simulink model "gm_sampleModel66206_pp_7_1_sub"  (R2023b)
settings: Solver=VariableStepAuto  StartTime=0.0  StopTime=10.0  RelTol=1e-3
libraries: simulink x38, hdlsllib x2, hdlmdlgenlib x2
(part 1 of 2)
settings Model: Creator=CW  LastModifiedBy=CW
settings OptimizationCC: BlockReduction=off  ConditionallyExecuteInputs=off
settings DebuggingCC: ArtificialAlgebraicLoopMsg=none  InheritedTsInSrcMsg=none

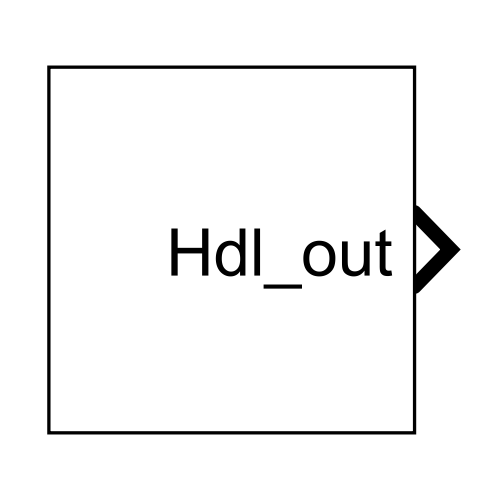
[thumbnail: Simulink's stored preview of the top-level diagram]
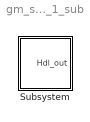
== system gm_sampleModel66206_pp_7_1_sub ==
  Subsystem : Subsystem

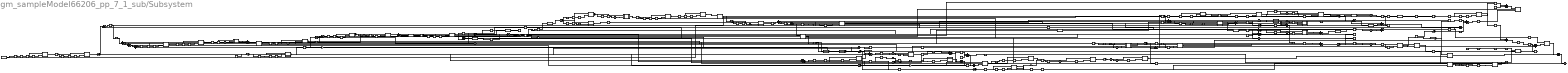
== system gm_sampleModel66206_pp_7_1_sub/Subsystem ==
  Reshape{,1..5} (6 alike) : Reshape
  cfblk1 : Subsystem  mask(Detect Fall Nonpositive){vinit=double(0), InputProcessing=Elements as channels (sample based), OutDataTypeStr=uint8}
      mask prompts: vinit "Simulink:masks:InitialCondition_MP"; InputProcessing "Simulink:masks:InputProcessing_MP"; OutDataTypeStr "Simulink:masks:OutputDataType_MP"
      mask help: Simulink:masks:DetectFallNonpositive_MD
      mask init:
      | InputProcessing = 'Elements as channels (sample based)';
      | OutDataTypeStr = 'uint8';
      | vinit = double(0);
      mask TypeOptions InputProcessing: Simulink:masks:ColumnsAsChannelsFrameBased | Simulink:masks:ElementsAsChannelsSampleBased
      mask TypeOptions OutDataTypeStr: Simulink:masks:uint8 | Simulink:masks:boolean
      mask Display: fprintf('U <= 0\n&  NOT\nU/z <= 0')
  cfblk10 : Subsystem  mask(Detect Rise Positive){vinit=double(0), InputProcessing=Elements as channels (sample based), OutDataTypeStr=uint8}
      mask prompts: vinit "Simulink:masks:InitialCondition_MP"; InputProcessing "Simulink:masks:InputProcessing_MP"; OutDataTypeStr "Simulink:masks:OutputDataType_MP"
      mask help: Simulink:masks:DetectRisePositive_MD
      mask init:
      | InputProcessing = 'Elements as channels (sample based)';
      | OutDataTypeStr = 'uint8';
      | vinit = double(0);
      mask TypeOptions InputProcessing: Simulink:masks:ColumnsAsChannelsFrameBased | Simulink:masks:ElementsAsChannelsSampleBased
      mask TypeOptions OutDataTypeStr: Simulink:masks:uint8 | Simulink:masks:boolean
      mask Display: fprintf('U > 0\n&  NOT\nU/z > 0')
  cfblk{15,22,25,48,52,58,61,63,68,71,90,98..100,106,113,115,118,129,134} (20 alike) : Sum  OutDataTypeStr=uint8  AccumDataTypeStr=uint8  SampleTime=1
  cfblk101 : Subsystem
  cfblk102_inst : Subsystem
  cfblk{29,37,41,46,67,76,93,103,116} (9 alike) : Sum  Inputs=+-  OutDataTypeStr=uint8  AccumDataTypeStr=uint8  SampleTime=1
  cfblk{16,33..34,73,82,91,97,105,121} (9 alike) : Gain  Gain="fi(0,0,8,7,\"hex\",\"80\")"  ParamDataTypeStr=fixdt(0, 8, 7)  OutDataTypeStr=uint8  SampleTime=1
  cfblk{18,79,107,109,125,140..141} (7 alike) : Product  Inputs=*/  OutDataTypeStr=uint8  RndMeth=Zero  SaturateOnIntegerOverflow=on  SampleTime=1
  cfblk108 : Subsystem
  cfblk11 : Subsystem  mask(Detect Fall Nonpositive){vinit=double(0), InputProcessing=Elements as channels (sample based), OutDataTypeStr=uint8}
      mask prompts: vinit "Simulink:masks:InitialCondition_MP"; InputProcessing "Simulink:masks:InputProcessing_MP"; OutDataTypeStr "Simulink:masks:OutputDataType_MP"
      mask help: Simulink:masks:DetectFallNonpositive_MD
      mask init:
      | InputProcessing = 'Elements as channels (sample based)';
      | OutDataTypeStr = 'uint8';
      | vinit = double(0);
      mask TypeOptions InputProcessing: Simulink:masks:ColumnsAsChannelsFrameBased | Simulink:masks:ElementsAsChannelsSampleBased
      mask TypeOptions OutDataTypeStr: Simulink:masks:uint8 | Simulink:masks:boolean
      mask Display: fprintf('U <= 0\n&  NOT\nU/z <= 0')
  cfblk{17,23,38..39,81,83,110,119,132} (9 alike) : ComplexToRealImag  SampleTime=1
  cfblk111 : Subsystem  mask(Real World Value Increment){}
      mask help: Simulink:masks:RealWorldValueIncrement_MD
      mask Display: disp('V++')
  cfblk{49,53,75,89,112,120,133} (7 alike) : Signum  SampleTime=1
  cfblk{60,69,85,114} (4 alike) : Sum  OutDataTypeStr=uint8  AccumDataTypeStr=uint8  RndMeth=Nearest  SampleTime=1
  cfblk114_const_val : Constant  Value=0  VectorParams1D=off  OutDataTypeStr=uint8  SampleTime=1
  cfblk117 : Subsystem
  cfblk12 : RelationalOperator  Operator=<=  OutDataTypeStr=fixdt(0,8,0)  SampleTime=1  InputSameDT=off
  cfblk122 : MinMax  OutDataTypeStr=uint8
  cfblk123 : Subsystem
  cfblk{56,65,124,139} (4 alike) : Abs  SampleTime=1  OutDataTypeStr=uint8  SaturateOnIntegerOverflow=off
  cfblk126 : MinMax  OutDataTypeStr=uint8
  cfblk{64,88,95,127,137} (5 alike) : Sum  Inputs=+  OutDataTypeStr=uint8
  cfblk128_inst : Subsystem
  cfblk13 : Subsystem
  cfblk130 : Subsystem
  cfblk131_inst : Subsystem
  cfblk135_inst : Subsystem
  cfblk136 : Subsystem
  cfblk138 : Subsystem
  cfblk14 : Subsystem
  cfblk143 : Constant  Value=0  VectorParams1D=off  OutDataTypeStr=uint8  SampleTime=1
  cfblk144 : Constant  Value=0  VectorParams1D=off  OutDataTypeStr=uint8  SampleTime=1
  cfblk145 : hdlsllib/Sources/HDL Counter  CountType=Count limited  CountInit=0  CountStep=1  CountMax=25  CountFromType=Initial value  CountFrom=0  CountResetPort=off  CountLoadPort=off  CountEnbPort=off  CountDirPort=off  CountHitOutputPort=off  CountDataType=Unsigned  CountWordLen=8  CountFracLen=0  CountSampTime=1
  cfblk146 : Subsystem
  cfblk147 : Subsystem
  cfblk148 : Subsystem
  cfblk149 : Subsystem
  cfblk150 : Subsystem
  cfblk151 : Subsystem
  cfblk{152..155} (4 alike) : Switch  Threshold=double(0)  OutDataTypeStr=uint8  SampleTime=1  SaturateOnIntegerOverflow=off  InputSameDT=off
  cfblk{156..167,169..174} (18 alike) : Delay  DelayLength=double(2)  InitialCondition=0  SampleTime=1
  cfblk168 : Subsystem
  cfblk{175..179,182..189,191,194..198} (19 alike) : DataTypeConversion  OutDataTypeStr=fixdt(0,8,0)
  cfblk180 : Subsystem
  cfblk181 : Subsystem
  cfblk19 : Subsystem  mask(Real World Value Increment){}
      mask help: Simulink:masks:RealWorldValueIncrement_MD
      mask Display: disp('V++')
  cfblk190 : Subsystem
  cfblk192 : Subsystem
  cfblk193 : Subsystem
  cfblk2 : Subsystem
  cfblk20_inst : Subsystem
  cfblk21 : Subsystem
  cfblk24 : Subsystem
  cfblk26 : Subsystem
  cfblk27 : Subsystem
  cfblk28 : Subsystem
  cfblk3 : RelationalOperator  Operator=<=  OutDataTypeStr=fixdt(0,8,0)  SampleTime=1  InputSameDT=off
  cfblk30_inst : Subsystem
  cfblk32 : Subsystem
  cfblk35 : Subsystem
  cfblk36_inst : Subsystem
  cfblk4 : hdlmdlgenlib/Buffer
  cfblk40 : Subsystem  mask(Real World Value Increment){}
      mask help: Simulink:masks:RealWorldValueIncrement_MD
      mask Display: disp('V++')
  cfblk42_inst : Subsystem
  cfblk44_inst : Subsystem
  cfblk47 : Subsystem
  cfblk5 : Subsystem
  cfblk50 : Subsystem
  cfblk51 : Subsystem
  cfblk54 : Subsystem
  cfblk55 : Subsystem
  cfblk59 : Subsystem  mask(Real World Value Increment){}
      mask help: Simulink:masks:RealWorldValueIncrement_MD
      mask Display: disp('V++')
  cfblk6 : hdlsllib/Logic and Bit Operations/Bit Reduce  mode=AND
  cfblk60_const_val : Constant  Value=0  VectorParams1D=off  OutDataTypeStr=uint8  SampleTime=1
  cfblk66 : Sum  Inputs=+-  OutDataTypeStr=uint8  AccumDataTypeStr=int32  SampleTime=1
  cfblk69_const_val : Constant  Value=0  VectorParams1D=off  OutDataTypeStr=uint8  SampleTime=1
  cfblk7 : hdlmdlgenlib/Buffer
  cfblk70 : Subsystem
  cfblk72 : Subsystem
  cfblk74 : Subsystem
  cfblk77 : Sum  OutDataTypeStr=uint8  AccumDataTypeStr=fixdt(0, 32, 7)  SampleTime=1
  cfblk8 : simulink/Logic and Bit Operations/Bit Set  iBit=double(0)
  cfblk80 : Subsystem  mask(Real World Value Increment){}
      mask help: Simulink:masks:RealWorldValueIncrement_MD
      mask Display: disp('V++')
  cfblk84 : Subsystem
  cfblk85_const_val : Constant  Value=0  VectorParams1D=off  OutDataTypeStr=uint8  SampleTime=1
  cfblk87 : MinMax  OutDataTypeStr=uint8
  cfblk9 : simulink/Logic and Bit Operations/Detect Decrease  vinit=0.0  OutDataTypeStr=uint8
      settings: LibrarySourceBlock=|
      | hdlsllib/Logic and Bit
      | Operations/Detect
      | Decrease
  cfblk92 : Subsystem
  cfblk94_inst : Subsystem
  cfblk96 : Subsystem
  compare{,4,6..7,10..12,15..16,18,20,24..34} (22 alike) : simulink/Logic and Bit Operations/Compare To Constant  relop=>=  const=0  OutDataTypeStr=boolean
  compare{1,5,8,13..14,19,22} (7 alike) : simulink/Logic and Bit Operations/Compare To Constant  relop=>=  const=255  OutDataTypeStr=boolean
  compare{2..3,9,17,21,23} (6 alike) : simulink/Logic and Bit Operations/Compare To Constant  relop=>=  const=1  OutDataTypeStr=boolean
  emi_{7,15,23,31,39,47,55,63,71,79,87,95,103,111,119,127,135,143,151,159,175,183,191,199,215,223,232,240,249,257,265,273,281,289} (34 alike) : DataTypeConversion  OutDataTypeStr=fixdt(0,8,0)
  emi_{8,24,32,40,48,56,64,72,80,88,96,104,136,144,152,184,192,200,224,241,258,290} (22 alike) : Delay  DelayLength=double(2)  InitialCondition=0  SampleTime=1
  emi_{16,112,160,208,216,250,274} (7 alike) : Delay  DelayLength=double(2)  InitialCondition=255  SampleTime=1
  emi_{120,128,176,233,266,282} (6 alike) : Delay  DelayLength=double(2)  InitialCondition=1  SampleTime=1
  emi_207 : DataTypeConversion  OutDataTypeStr=uint8  SampleTime=1  SaturateOnIntegerOverflow=off  RndMeth=Floor
  Hdl_out : Outport  OutDataTypeStr=uint8  SampleTime=1
  wires:
  cfblk1/1(Y) -> cfblk198/1
  cfblk10/1(Y) -> cfblk83/1
  cfblk100/1 -> emi_16/1, cfblk117/1(emi_10)
  cfblk101/1(emi_67) -> emi_88/1, cfblk84/1(emi_82)
  cfblk102_inst/1(out1) -> cfblk66/1, cfblk134/2
  cfblk103/1 -> emi_290/1, cfblk96/1(emi_284)
  Reshape/1 -> cfblk155/3, emi_192/1, cfblk47/1(emi_186)
  cfblk105/1 -> cfblk155/1
  cfblk106/1 -> cfblk76/1
  cfblk107/1 -> emi_64/1, cfblk14/1(emi_58)
  cfblk108/1(emi_2) -> cfblk49/1
  cfblk108/2(emi_3) -> cfblk97/1
  cfblk109/1 -> cfblk166/1
  cfblk11/1(Y) -> cfblk157/1
  cfblk110/1 -> cfblk56/1
  cfblk110/2 -> cfblk48/1
  cfblk111/1(y) -> cfblk89/1
  cfblk112/1 -> emi_48/1, cfblk136/1(emi_42)
  cfblk113/1 -> cfblk153/3, cfblk135_inst/1(in1)
  cfblk114/1 -> emi_250/1, cfblk70/1(emi_243)
  cfblk115/1 -> cfblk134/1
  cfblk116/1 -> cfblk19/1(u)
  cfblk117/1(emi_11) -> cfblk37/1
  cfblk118/1 -> cfblk184/1
  cfblk119/1 -> cfblk73/1
  cfblk119/2 -> cfblk132/1
  cfblk12/1 -> cfblk179/1
  cfblk120/1 -> cfblk63/1, cfblk161/1
  cfblk121/1 -> cfblk186/1, cfblk141/2
  cfblk122/1 -> cfblk11/1(U)
  cfblk123/1(emi_19) -> cfblk77/1
  cfblk124/1 -> cfblk60/1, cfblk100/2, cfblk165/1
  cfblk125/1 -> cfblk116/1, cfblk10/1(U)
  cfblk126/1 -> cfblk195/1
  cfblk127/1 -> cfblk90/1
  cfblk128_inst/1(out1) -> cfblk81/1
  cfblk129/1 -> cfblk163/1
  cfblk13/1(emi_27) -> cfblk113/1
  cfblk130/1(emi_35) -> cfblk53/1
  cfblk131_inst/1(out1) -> cfblk22/2
  cfblk132/1 -> cfblk80/1(u)
  cfblk132/2 -> cfblk167/1
  cfblk133/1 -> cfblk188/1, cfblk174/1
  cfblk134/1 -> emi_72/1, cfblk101/1(emi_66)
  cfblk135_inst/1(out1) -> emi_136/1, cfblk24/1(emi_130)
  cfblk136/1(emi_43) -> Reshape2/1, cfblk41/2
  cfblk137/1 -> cfblk93/2, emi_56/1, cfblk138/1(emi_50)
  cfblk138/1(emi_51) -> cfblk61/2
  cfblk139/1 -> Reshape4/1, cfblk105/1
  cfblk14/1(emi_59) -> cfblk15/2
  cfblk140/1 -> emi_112/1, cfblk192/1(emi_106)
  cfblk141/1 -> cfblk185/1
  cfblk143/1 -> cfblk196/1, cfblk34/1
  cfblk144/1 -> cfblk182/1
  cfblk145/1 -> Reshape/1
  cfblk146/1(Out1) -> cfblk112/1
  cfblk147/1(Out1) -> cfblk175/1
  cfblk148/1(Out1) -> cfblk40/1(u), cfblk64/1
  cfblk149/1(Out1) -> cfblk124/1
  cfblk15/1 -> cfblk158/1
  cfblk150/1(Out1) -> cfblk58/1
  cfblk151/1(Out1) -> cfblk110/1
  cfblk152/1 -> cfblk102_inst/2(in2)
  cfblk153/1 -> cfblk68/2, cfblk122/1
  cfblk154/1 -> cfblk103/2
  cfblk155/1 -> cfblk12/2
  cfblk156/1 -> cfblk116/2
  cfblk157/1 -> cfblk153/2
  cfblk158/1 -> cfblk115/2
  cfblk159/1 -> cfblk152/2
  cfblk16/1 -> cfblk68/1, cfblk67/1
  cfblk160/1 -> cfblk113/2
  cfblk161/1 -> cfblk135_inst/2(in2)
  cfblk162/1 -> cfblk41/1
  cfblk163/1 -> cfblk76/2
  cfblk164/1 -> cfblk141/1
  cfblk165/1 -> cfblk67/2
  cfblk166/1 -> cfblk61/1
  cfblk167/1 -> cfblk71/1
  cfblk168/1(emi_91) -> cfblk125/1
  cfblk169/1 -> cfblk152/3
  cfblk17/1 -> cfblk121/1
  cfblk17/2 -> cfblk9/1
  cfblk170/1 -> cfblk154/2
  cfblk171/1 -> cfblk106/2
  cfblk172/1 -> cfblk20_inst/1(in1)
  cfblk173/1 -> cfblk128_inst/2(in2)
  cfblk174/1 -> cfblk1/1(U)
  cfblk175/1 -> emi_282/1, emi_176/1, cfblk92/1(emi_276), cfblk32/1(emi_170)
  cfblk176/1 -> cfblk147/1(In1)
  cfblk177/1 -> cfblk120/1
  cfblk178/1 -> cfblk99/1
  cfblk179/1 -> cfblk99/2
  cfblk18/1 -> emi_274/1, cfblk181/1(emi_268)
  cfblk180/1(emi_75) -> cfblk93/1, cfblk131_inst/2(in2), cfblk160/1
  cfblk181/1(emi_269) -> cfblk91/1
  cfblk182/1 -> cfblk8/1
  cfblk183/1 -> cfblk102_inst/1(in1)
  cfblk184/1 -> cfblk30_inst/2(in2)
  cfblk185/1 -> cfblk118/1
  cfblk186/1 -> cfblk118/2
  cfblk187/1 -> cfblk75/1
  cfblk188/1 -> cfblk59/1(u)
  cfblk189/1 -> cfblk44_inst/1(in1)
  cfblk19/1(y) -> cfblk71/2
  cfblk190/1(emi_99) -> cfblk25/1
  cfblk191/1 -> cfblk25/2
  cfblk192/1(emi_107) -> emi_160/1, cfblk28/1(emi_154)
  cfblk193/1(emi_115) -> cfblk140/1
  cfblk194/1 -> cfblk140/2
  cfblk195/1 -> cfblk107/1
  cfblk196/1 -> cfblk126/1
  cfblk197/1 -> emi_266/1, cfblk74/1(emi_260)
  cfblk198/1 -> emi_224/1, cfblk51/1(emi_218)
  cfblk2/1(emi_195) -> cfblk18/1
  cfblk20_inst/1(out1) -> emi_184/1, cfblk35/1(emi_178)
  cfblk21/1(emi_123) -> Reshape5/1
  cfblk22/1 -> cfblk162/1
  cfblk23/1 -> cfblk29/2
  cfblk23/2 -> cfblk69/1
  cfblk24/1(emi_131) -> cfblk154/3, cfblk95/1
  cfblk25/1 -> cfblk189/1
  cfblk26/1(emi_139) -> cfblk137/1
  cfblk27/1(emi_147) -> cfblk129/1
  cfblk28/1(emi_155) -> cfblk36_inst/1(in1)
  cfblk29/1 -> cfblk146/1(In1)
  cfblk3/1 -> cfblk176/1
  cfblk30_inst/1(out1) -> cfblk154/1
  cfblk32/1(emi_171) -> cfblk164/1
  cfblk33/1 -> cfblk12/1
  cfblk34/1 -> cfblk94_inst/1(in1)
  cfblk35/1(emi_179) -> cfblk152/1
  cfblk36_inst/1(out1) -> Reshape1/1
  cfblk37/1 -> cfblk111/1(u)
  cfblk38/1 -> cfblk88/1
  cfblk38/2 -> cfblk194/1, cfblk173/1
  cfblk39/1 -> cfblk33/1
  cfblk39/2 -> cfblk3/1
  cfblk4/1 -> cfblk6/1, cfblk125/2
  cfblk40/1(y) -> cfblk65/1, cfblk155/2
  cfblk41/1 -> cfblk153/1, cfblk170/1, cfblk151/1(In1)
  cfblk42_inst/1(out1) -> cfblk172/1
  cfblk44_inst/1(out1) -> cfblk22/1
  Reshape1/1 -> emi_40/1, cfblk130/1(emi_34)
  cfblk46/1 -> cfblk39/1
  cfblk47/1(emi_187) -> cfblk98/2, cfblk63/2, cfblk139/1
  cfblk48/1 -> cfblk46/1
  cfblk49/1 -> cfblk169/1
  cfblk5/1(emi_203) -> cfblk87/1
  cfblk50/1(emi_211) -> emi_208/1, cfblk5/1(emi_202)
  cfblk51/1(emi_219) -> cfblk197/1
  cfblk52/1 -> cfblk109/1
  cfblk53/1 -> cfblk129/2
  cfblk54/1(emi_227) -> cfblk178/1
  cfblk54/2(emi_228) -> cfblk23/1
  cfblk55/1(emi_236) -> cfblk42_inst/2(in2), cfblk17/1
  cfblk56/1 -> cfblk90/2, cfblk107/2
  Reshape2/1 -> cfblk156/1
  cfblk58/1 -> cfblk119/1
  cfblk59/1(y) -> cfblk187/1
  cfblk6/1 -> cfblk66/2
  cfblk60/1 -> cfblk37/2, cfblk3/2
  cfblk61/1 -> cfblk38/1
  Reshape3/1 -> cfblk85/1
  cfblk63/1 -> cfblk44_inst/2(in2)
  cfblk64/1 -> cfblk20_inst/2(in2)
  cfblk65/1 -> cfblk77/2, Hdl_out/1
  cfblk66/1 -> cfblk115/1, cfblk109/2
  cfblk67/1 -> cfblk4/1
  cfblk68/1 -> emi_24/1, cfblk82/1, cfblk123/1(emi_18)
  cfblk69/1 -> cfblk30_inst/1(in1)
  cfblk7/1 -> cfblk100/1
  cfblk70/1(emi_244) -> cfblk149/1(In1)
  cfblk70/2(emi_245) -> cfblk58/2
  cfblk71/1 -> cfblk106/1
  cfblk72/1(emi_253) -> cfblk29/1
  cfblk73/1 -> cfblk52/2, emi_152/1, cfblk27/1(emi_146)
  cfblk74/1(emi_261) -> cfblk16/1
  cfblk75/1 -> cfblk36_inst/2(in2), emi_233/1, cfblk54/1(emi_226)
  cfblk76/1 -> cfblk7/1, cfblk128_inst/1(in1), emi_104/1, cfblk190/1(emi_98)
  cfblk77/1 -> emi_128/1, cfblk21/1(emi_122)
  Reshape4/1 -> cfblk103/1
  cfblk79/1 -> cfblk114/1, emi_216/1, cfblk50/1(emi_210)
  cfblk8/1 -> cfblk183/1
  cfblk80/1(y) -> cfblk52/1
  cfblk81/1 -> cfblk148/1(In1)
  cfblk81/2 -> cfblk42_inst/1(in1), cfblk150/1(In1)
  cfblk82/1 -> emi_8/1, cfblk108/1(emi_1)
  cfblk83/1 -> cfblk79/2
  cfblk83/2 -> cfblk133/1
  cfblk84/1(emi_83) -> cfblk46/2, emi_32/1, cfblk13/1(emi_26)
  cfblk85/1 -> cfblk98/1, cfblk159/1
  Reshape5/1 -> cfblk127/1
  cfblk87/1 -> emi_96/1, cfblk168/1(emi_90)
  cfblk88/1 -> emi_241/1, cfblk55/1(emi_235)
  cfblk89/1 -> cfblk48/2, cfblk191/1
  cfblk9/1 -> cfblk131_inst/1(in1), cfblk171/1
  cfblk90/1 -> Reshape3/1, cfblk15/1
  cfblk91/1 -> emi_80/1, cfblk180/1(emi_74)
  cfblk92/1(emi_277) -> emi_120/1, cfblk193/1(emi_114)
  cfblk93/1 -> cfblk79/1
  cfblk94_inst/1(out1) -> emi_200/1, cfblk2/1(emi_194)
  cfblk95/1 -> emi_144/1, cfblk26/1(emi_138)
  cfblk96/1(emi_285) -> emi_258/1, cfblk72/1(emi_252)
  cfblk97/1 -> cfblk18/2
  cfblk98/1 -> cfblk94_inst/2(in2)
  cfblk99/1 -> cfblk177/1
  emi_103/1 -> compare/1
  emi_104/1 -> emi_103/1
  emi_111/1 -> compare1/1
  emi_112/1 -> emi_111/1
  emi_119/1 -> compare2/1
  emi_120/1 -> emi_119/1
  emi_127/1 -> compare3/1
  emi_128/1 -> emi_127/1
  emi_135/1 -> compare4/1
  emi_136/1 -> emi_135/1
  emi_143/1 -> compare6/1
  emi_144/1 -> emi_143/1
  emi_15/1 -> compare5/1
  emi_151/1 -> compare7/1
  emi_152/1 -> emi_151/1
  emi_159/1 -> compare8/1
  emi_16/1 -> emi_15/1
  emi_160/1 -> emi_159/1
  emi_175/1 -> compare9/1
  emi_176/1 -> emi_175/1
  emi_183/1 -> compare10/1
  emi_184/1 -> emi_183/1
  emi_191/1 -> compare11/1
  emi_192/1 -> emi_191/1
  emi_199/1 -> compare12/1
  emi_200/1 -> emi_199/1
  emi_207/1 -> compare13/1
  emi_208/1 -> emi_207/1
  emi_215/1 -> compare14/1
  emi_216/1 -> emi_215/1
  emi_223/1 -> compare16/1
  emi_224/1 -> emi_223/1
  emi_23/1 -> compare15/1
  emi_232/1 -> compare17/1
  emi_233/1 -> emi_232/1
  emi_24/1 -> emi_23/1
  emi_240/1 -> compare18/1
  emi_241/1 -> emi_240/1
  emi_249/1 -> compare19/1
  emi_250/1 -> emi_249/1
  emi_257/1 -> compare20/1
  emi_258/1 -> emi_257/1
  emi_265/1 -> compare21/1
  emi_266/1 -> emi_265/1
  emi_273/1 -> compare22/1
  emi_274/1 -> emi_273/1
  emi_281/1 -> compare23/1
  emi_282/1 -> emi_281/1
  emi_289/1 -> compare24/1
  emi_290/1 -> emi_289/1
  emi_31/1 -> compare25/1
  emi_32/1 -> emi_31/1
  emi_39/1 -> compare26/1
  emi_40/1 -> emi_39/1
  emi_47/1 -> compare27/1
  emi_48/1 -> emi_47/1
  emi_55/1 -> compare28/1
  emi_56/1 -> emi_55/1
  emi_63/1 -> compare30/1
  emi_64/1 -> emi_63/1
  emi_7/1 -> compare29/1
  emi_71/1 -> compare31/1
  emi_72/1 -> emi_71/1
  emi_79/1 -> compare32/1
  emi_8/1 -> emi_7/1
  emi_80/1 -> emi_79/1
  emi_87/1 -> compare33/1
  emi_88/1 -> emi_87/1
  emi_95/1 -> compare34/1
  emi_96/1 -> emi_95/1
  cfblk114_const_val/1 -> cfblk114/2
  cfblk60_const_val/1 -> cfblk60/2
  cfblk69_const_val/1 -> cfblk69/2
  cfblk85_const_val/1 -> cfblk85/2
  compare/1 -> cfblk190/2(Action Port)
  compare1/1 -> cfblk192/2(Action Port)
  compare2/1 -> cfblk193/2(Action Port)
  compare3/1 -> cfblk21/2(Action Port)
  compare4/1 -> cfblk24/2(Action Port)
  compare5/1 -> cfblk117/2(Action Port)
  compare6/1 -> cfblk26/2(Action Port)
  compare7/1 -> cfblk27/2(Action Port)
  compare8/1 -> cfblk28/2(Action Port)
  compare9/1 -> cfblk32/2(Action Port)
  compare10/1 -> cfblk35/2(Action Port)
  compare11/1 -> cfblk47/2(Action Port)
  compare12/1 -> cfblk2/2(Action Port)
  compare13/1 -> cfblk5/2(Action Port)
  compare14/1 -> cfblk50/2(Action Port)
  compare15/1 -> cfblk123/2(Action Port)
  compare16/1 -> cfblk51/2(Action Port)
  compare17/1 -> cfblk54/2(Action Port)
  compare18/1 -> cfblk55/2(Action Port)
  compare19/1 -> cfblk70/2(Action Port)
  compare20/1 -> cfblk72/2(Action Port)
  compare21/1 -> cfblk74/2(Action Port)
  compare22/1 -> cfblk181/2(Action Port)
  compare23/1 -> cfblk92/2(Action Port)
  compare24/1 -> cfblk96/2(Action Port)
  compare25/1 -> cfblk13/2(Action Port)
  compare26/1 -> cfblk130/2(Action Port)
  compare27/1 -> cfblk136/2(Action Port)
  compare28/1 -> cfblk138/2(Action Port)
  compare29/1 -> cfblk108/2(Action Port)
  compare30/1 -> cfblk14/2(Action Port)
  compare31/1 -> cfblk101/2(Action Port)
  compare32/1 -> cfblk180/2(Action Port)
  compare33/1 -> cfblk84/2(Action Port)
  compare34/1 -> cfblk168/2(Action Port)

== system gm_sampleModel66206_pp_7_1_sub/Subsystem/cfblk1 ==
  note: U(k)
  note: Edge
  U : Inport  OutDataTypeStr=uint8  SampleTime=1
  Delay Input1 : UnitDelay  Description=Store in Global RAM  DisableCoverage=on  InitialCondition=vinit  SampleTime=-1  HasFrameUpgradeWarning=on
  FixPt Relational Operator : RelationalOperator  Operator=>  OutDataTypeStr=fixdt(0, 8)  ZeroCross=off  InputSameDT=off
  Nonpositive : Subsystem  mask(Compare To Zero){relop=<=, OutDataTypeStr=boolean, ZeroCross=off}
      mask prompts: relop "Simulink:masks:Operator_MP"; OutDataTypeStr "Simulink:masks:OutputDataType_MP"; ZeroCross "Simulink:masks:EnableZerocrossingDetection_MP"
      mask help: Simulink:masks:CompareToZero_MD
      mask init:
      | OutDataTypeStr = 'boolean';
      | ZeroCross = 'off';
      | blkName = 'sampleModel66206_pp_7_1_sub/Subsystem/cfblk1/Nonpositive';
      | relop = '<=';
      | setValue = 'boolean';
      mask TypeOptions relop: == | ~= | < | <= | >= | >
      mask TypeOptions OutDataTypeStr: Simulink:masks:uint8 | Simulink:masks:boolean
      mask Callback ZeroCross: sl('zeroCrossEnable', gcbh);
      mask Display: disp([relop,' 0'])
  Y : Outport  SampleTime=1
  wires:
  U/1 -> Nonpositive/1(u)
  Delay Input1/1 -> FixPt Relational Operator/2
  FixPt Relational Operator/1 -> Y/1
  Nonpositive/1(y) -> FixPt Relational Operator/1, Delay Input1/1

== system gm_sampleModel66206_pp_7_1_sub/Subsystem/cfblk10 ==
  note: U(k)
  note: Edge
  U : Inport  OutDataTypeStr=uint8  SampleTime=1
  Delay Input1 : UnitDelay  Description=Store in Global RAM  DisableCoverage=on  InitialCondition=vinit  SampleTime=-1  HasFrameUpgradeWarning=on
  FixPt Relational Operator : RelationalOperator  Operator=>  OutDataTypeStr=fixdt(0, 8)  ZeroCross=off  InputSameDT=off
  Positive : Subsystem  mask(Compare To Zero){relop=>, OutDataTypeStr=boolean, ZeroCross=off}
      mask prompts: relop "Simulink:masks:Operator_MP"; OutDataTypeStr "Simulink:masks:OutputDataType_MP"; ZeroCross "Simulink:masks:EnableZerocrossingDetection_MP"
      mask help: Simulink:masks:CompareToZero_MD
      mask init:
      | OutDataTypeStr = 'boolean';
      | ZeroCross = 'off';
      | blkName = 'sampleModel66206_pp_7_1_sub/Subsystem/cfblk10/Positive';
      | relop = '>';
      | setValue = 'boolean';
      mask TypeOptions relop: == | ~= | < | <= | >= | >
      mask TypeOptions OutDataTypeStr: Simulink:masks:uint8 | Simulink:masks:boolean
      mask Callback ZeroCross: sl('zeroCrossEnable', gcbh);
      mask Display: disp([relop,' 0'])
  Y : Outport  SampleTime=1
  wires:
  U/1 -> Positive/1(u)
  Delay Input1/1 -> FixPt Relational Operator/2
  FixPt Relational Operator/1 -> Y/1
  Positive/1(y) -> FixPt Relational Operator/1, Delay Input1/1

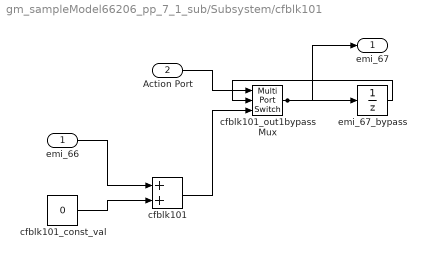
== system gm_sampleModel66206_pp_7_1_sub/Subsystem/cfblk101 ==
  emi_66 : Inport  OutDataTypeStr=uint8  PortDimensions=1  SampleTime=1
  Action Port : Inport  Port=2  OutDataTypeStr=boolean  SampleTime=1
  cfblk101 : Sum  OutDataTypeStr=uint8  AccumDataTypeStr=uint8  RndMeth=Nearest  SampleTime=1
  cfblk101_const_val : Constant  Value=0  VectorParams1D=off  OutDataTypeStr=uint8  SampleTime=1
  cfblk101_out1bypassMux : MultiPortSwitch  DataPortOrder=Zero-based contiguous  Inputs=2  zeroidx=on  OutDataTypeStr=uint8  SampleTime=1  SaturateOnIntegerOverflow=off  InputSameDT=off
  emi_67_bypass : UnitDelay  InitialCondition="fi(0,0,8,0,\"hex\",\"00\")"  SampleTime=1
  emi_67 : Outport  SampleTime=1  InitialOutput=0
  wires:
  Action Port/1 -> cfblk101_out1bypassMux/1
  emi_66/1 -> cfblk101/1
  cfblk101/1 -> cfblk101_out1bypassMux/3
  cfblk101_out1bypassMux/1 -> emi_67_bypass/1, emi_67/1
  emi_67_bypass/1 -> cfblk101_out1bypassMux/2
  cfblk101_const_val/1 -> cfblk101/2

== system gm_sampleModel66206_pp_7_1_sub/Subsystem/cfblk102_inst ==
  in1 : Inport  OutDataTypeStr=uint8  SampleTime=1
  in2 : Inport  Port=2  OutDataTypeStr=uint8  SampleTime=1
  mul_cfblk102_dotp_mulcomp : Product  Inputs=**  OutDataTypeStr=uint8  SampleTime=1
  out1 : Outport  OutDataTypeStr=uint8  SampleTime=1
  wires:
  in1/1 -> mul_cfblk102_dotp_mulcomp/1
  in2/1 -> mul_cfblk102_dotp_mulcomp/2
  mul_cfblk102_dotp_mulcomp/1 -> out1/1

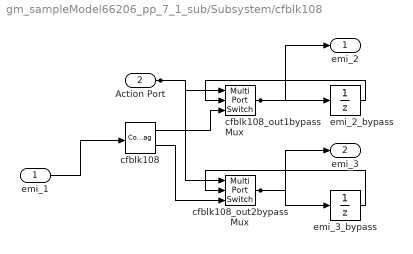
== system gm_sampleModel66206_pp_7_1_sub/Subsystem/cfblk108 ==
  emi_1 : Inport  OutDataTypeStr=uint8  PortDimensions=1  SampleTime=1
  Action Port : Inport  Port=2  OutDataTypeStr=boolean  SampleTime=1
  cfblk108 : ComplexToRealImag  SampleTime=1
  cfblk108_out1bypassMux : MultiPortSwitch  DataPortOrder=Zero-based contiguous  Inputs=2  zeroidx=on  OutDataTypeStr=uint8  SampleTime=1  SaturateOnIntegerOverflow=off  InputSameDT=off
  cfblk108_out2bypassMux : MultiPortSwitch  DataPortOrder=Zero-based contiguous  Inputs=2  zeroidx=on  OutDataTypeStr=uint8  SampleTime=1  SaturateOnIntegerOverflow=off  InputSameDT=off
  emi_2_bypass : UnitDelay  InitialCondition="fi(0,0,8,0,\"hex\",\"00\")"  SampleTime=1
  emi_3_bypass : UnitDelay  InitialCondition="fi(0,0,8,0,\"hex\",\"00\")"  SampleTime=1
  emi_2 : Outport  SampleTime=1  InitialOutput=0
  emi_3 : Outport  Port=2  SampleTime=1  InitialOutput=0
  wires:
  Action Port/1 -> cfblk108_out2bypassMux/1, cfblk108_out1bypassMux/1
  emi_1/1 -> cfblk108/1
  cfblk108/1 -> cfblk108_out1bypassMux/3
  cfblk108/2 -> cfblk108_out2bypassMux/3
  cfblk108_out1bypassMux/1 -> emi_2_bypass/1, emi_2/1
  emi_2_bypass/1 -> cfblk108_out1bypassMux/2
  cfblk108_out2bypassMux/1 -> emi_3_bypass/1, emi_3/1
  emi_3_bypass/1 -> cfblk108_out2bypassMux/2

== system gm_sampleModel66206_pp_7_1_sub/Subsystem/cfblk11 ==
  note: U(k)
  note: Edge
  U : Inport  OutDataTypeStr=uint8  SampleTime=1
  Delay Input1 : UnitDelay  Description=Store in Global RAM  DisableCoverage=on  InitialCondition=vinit  SampleTime=-1  HasFrameUpgradeWarning=on
  FixPt Relational Operator : RelationalOperator  Operator=>  OutDataTypeStr=fixdt(0, 8)  ZeroCross=off  InputSameDT=off
  Nonpositive : Subsystem  mask(Compare To Zero){relop=<=, OutDataTypeStr=boolean, ZeroCross=off}
      mask prompts: relop "Simulink:masks:Operator_MP"; OutDataTypeStr "Simulink:masks:OutputDataType_MP"; ZeroCross "Simulink:masks:EnableZerocrossingDetection_MP"
      mask help: Simulink:masks:CompareToZero_MD
      mask init:
      | OutDataTypeStr = 'boolean';
      | ZeroCross = 'off';
      | blkName = 'sampleModel66206_pp_7_1_sub/Subsystem/cfblk11/Nonpositive';
      | relop = '<=';
      | setValue = 'boolean';
      mask TypeOptions relop: == | ~= | < | <= | >= | >
      mask TypeOptions OutDataTypeStr: Simulink:masks:uint8 | Simulink:masks:boolean
      mask Callback ZeroCross: sl('zeroCrossEnable', gcbh);
      mask Display: disp([relop,' 0'])
  Y : Outport  SampleTime=1
  wires:
  U/1 -> Nonpositive/1(u)
  Delay Input1/1 -> FixPt Relational Operator/2
  FixPt Relational Operator/1 -> Y/1
  Nonpositive/1(y) -> FixPt Relational Operator/1, Delay Input1/1

== system gm_sampleModel66206_pp_7_1_sub/Subsystem/cfblk111 ==
  u : Inport  OutDataTypeStr=uint8  SampleTime=1
  FixPt Constant : Constant  DisableCoverage=on  OutDataTypeStr=Inherit: Inherit via back propagation  SampleTime=-1
  FixPt Data Type Duplicate : DataTypeDuplicate  DisableCoverage=on  NumInputPorts=3
  FixPt Sum1 : Sum  OutDataTypeStr=Inherit: Inherit via back propagation  InputSameDT=on  LockScale=on
  y : Outport  SampleTime=1
  wires:
  u/1 -> FixPt Sum1/1, FixPt Data Type Duplicate/2
  FixPt Constant/1 -> FixPt Sum1/2, FixPt Data Type Duplicate/3
  FixPt Sum1/1 -> FixPt Data Type Duplicate/1, y/1

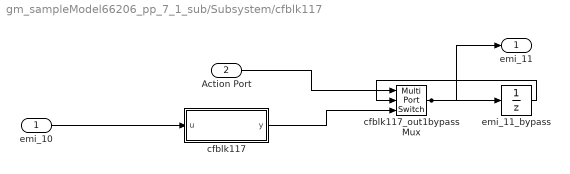
== system gm_sampleModel66206_pp_7_1_sub/Subsystem/cfblk117 ==
  emi_10 : Inport  OutDataTypeStr=uint8  PortDimensions=1  SampleTime=1
  Action Port : Inport  Port=2  OutDataTypeStr=boolean  SampleTime=1
  cfblk117 : Subsystem  mask(Real World Value Increment){}
      mask help: Simulink:masks:RealWorldValueIncrement_MD
      mask Display: disp('V++')
  cfblk117_out1bypassMux : MultiPortSwitch  DataPortOrder=Zero-based contiguous  Inputs=2  zeroidx=on  OutDataTypeStr=uint8  SampleTime=1  SaturateOnIntegerOverflow=off  InputSameDT=off
  emi_11_bypass : UnitDelay  InitialCondition="fi(0,0,8,0,\"hex\",\"00\")"  SampleTime=1
  emi_11 : Outport  SampleTime=1  InitialOutput=0
  wires:
  Action Port/1 -> cfblk117_out1bypassMux/1
  emi_10/1 -> cfblk117/1(u)
  cfblk117/1(y) -> cfblk117_out1bypassMux/3
  cfblk117_out1bypassMux/1 -> emi_11_bypass/1, emi_11/1
  emi_11_bypass/1 -> cfblk117_out1bypassMux/2

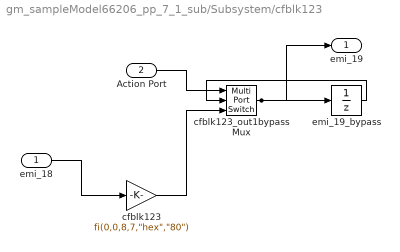
== system gm_sampleModel66206_pp_7_1_sub/Subsystem/cfblk123 ==
  emi_18 : Inport  OutDataTypeStr=uint8  PortDimensions=1  SampleTime=1
  Action Port : Inport  Port=2  OutDataTypeStr=boolean  SampleTime=1
  cfblk123 : Gain  Gain="fi(0,0,8,7,\"hex\",\"80\")"  ParamDataTypeStr=fixdt(0, 8, 7)  OutDataTypeStr=fixdt(0, 16, 7)  SampleTime=1
  cfblk123_out1bypassMux : MultiPortSwitch  DataPortOrder=Zero-based contiguous  Inputs=2  zeroidx=on  OutDataTypeStr=fixdt(0, 16, 7)  SampleTime=1  SaturateOnIntegerOverflow=off  InputSameDT=off
  emi_19_bypass : UnitDelay  InitialCondition="fi(0,0,16,7,\"hex\",\"0000\")"  SampleTime=1
  emi_19 : Outport  SampleTime=1  InitialOutput=0
  wires:
  Action Port/1 -> cfblk123_out1bypassMux/1
  emi_18/1 -> cfblk123/1
  cfblk123/1 -> cfblk123_out1bypassMux/3
  cfblk123_out1bypassMux/1 -> emi_19_bypass/1, emi_19/1
  emi_19_bypass/1 -> cfblk123_out1bypassMux/2

== system gm_sampleModel66206_pp_7_1_sub/Subsystem/cfblk128_inst ==
  in1 : Inport  OutDataTypeStr=uint8  SampleTime=1
  in2 : Inport  Port=2  OutDataTypeStr=uint8  SampleTime=1
  mul_cfblk128_dotp_mulcomp : Product  Inputs=**  OutDataTypeStr=uint8  SampleTime=1
  out1 : Outport  OutDataTypeStr=uint8  SampleTime=1
  wires:
  in1/1 -> mul_cfblk128_dotp_mulcomp/1
  in2/1 -> mul_cfblk128_dotp_mulcomp/2
  mul_cfblk128_dotp_mulcomp/1 -> out1/1

== system gm_sampleModel66206_pp_7_1_sub/Subsystem/cfblk13 ==
  emi_26 : Inport  OutDataTypeStr=uint8  PortDimensions=1  SampleTime=1
  Action Port : Inport  Port=2  OutDataTypeStr=boolean  SampleTime=1
  cfblk13 : Subsystem  mask(Detect Rise Nonnegative){vinit=double(0), InputProcessing=Elements as channels (sample based), OutDataTypeStr=uint8}
      mask prompts: vinit "Simulink:masks:InitialCondition_MP"; InputProcessing "Simulink:masks:InputProcessing_MP"; OutDataTypeStr "Simulink:masks:OutputDataType_MP"
      mask help: Simulink:masks:DetectRiseNonnegative_MD
      mask TypeOptions InputProcessing: Simulink:masks:ColumnsAsChannelsFrameBased | Simulink:masks:ElementsAsChannelsSampleBased
      mask TypeOptions OutDataTypeStr: Simulink:masks:uint8 | Simulink:masks:boolean
      mask Display: fprintf('U >= 0\n&  NOT\nU/z >= 0')
  cfblk13_out1bypassMux : MultiPortSwitch  DataPortOrder=Zero-based contiguous  Inputs=2  zeroidx=on  OutDataTypeStr=uint8  SampleTime=1  SaturateOnIntegerOverflow=off  InputSameDT=off
  emi_27_bypass : UnitDelay  InitialCondition="fi(0,0,8,0,\"hex\",\"00\")"  SampleTime=1
  emi_27 : Outport  SampleTime=1  InitialOutput=0
  wires:
  Action Port/1 -> cfblk13_out1bypassMux/1, cfblk13/2(Action Port_out2)
  emi_26/1 -> cfblk13/1(U)
  cfblk13/1(Y) -> cfblk13_out1bypassMux/3
  cfblk13_out1bypassMux/1 -> emi_27_bypass/1, emi_27/1
  emi_27_bypass/1 -> cfblk13_out1bypassMux/2

== system gm_sampleModel66206_pp_7_1_sub/Subsystem/cfblk130 ==
  emi_34 : Inport  OutDataTypeStr=uint8  PortDimensions=1  SampleTime=1
  Action Port : Inport  Port=2  OutDataTypeStr=boolean  SampleTime=1
  cfblk130 : Subsystem  mask(Real World Value Increment){}
      mask help: Simulink:masks:RealWorldValueIncrement_MD
      mask Display: disp('V++')
  cfblk130_out1bypassMux : MultiPortSwitch  DataPortOrder=Zero-based contiguous  Inputs=2  zeroidx=on  OutDataTypeStr=uint8  SampleTime=1  SaturateOnIntegerOverflow=off  InputSameDT=off
  emi_35_bypass : UnitDelay  InitialCondition="fi(0,0,8,0,\"hex\",\"00\")"  SampleTime=1
  emi_35 : Outport  SampleTime=1  InitialOutput=0
  wires:
  Action Port/1 -> cfblk130_out1bypassMux/1
  emi_34/1 -> cfblk130/1(u)
  cfblk130/1(y) -> cfblk130_out1bypassMux/3
  cfblk130_out1bypassMux/1 -> emi_35_bypass/1, emi_35/1
  emi_35_bypass/1 -> cfblk130_out1bypassMux/2

== system gm_sampleModel66206_pp_7_1_sub/Subsystem/cfblk131_inst ==
  in1 : Inport  OutDataTypeStr=uint8  SampleTime=1
  in2 : Inport  Port=2  OutDataTypeStr=uint8  SampleTime=1
  mul_cfblk131_dotp_mulcomp : Product  Inputs=**  OutDataTypeStr=uint8  SampleTime=1
  out1 : Outport  OutDataTypeStr=uint8  SampleTime=1
  wires:
  in1/1 -> mul_cfblk131_dotp_mulcomp/1
  in2/1 -> mul_cfblk131_dotp_mulcomp/2
  mul_cfblk131_dotp_mulcomp/1 -> out1/1

== system gm_sampleModel66206_pp_7_1_sub/Subsystem/cfblk135_inst ==
  in1 : Inport  OutDataTypeStr=uint8  SampleTime=1
  in2 : Inport  Port=2  OutDataTypeStr=uint8  SampleTime=1
  mul_cfblk135_dotp_mulcomp : Product  Inputs=**  OutDataTypeStr=uint8  SampleTime=1
  out1 : Outport  OutDataTypeStr=uint8  SampleTime=1
  wires:
  in1/1 -> mul_cfblk135_dotp_mulcomp/1
  in2/1 -> mul_cfblk135_dotp_mulcomp/2
  mul_cfblk135_dotp_mulcomp/1 -> out1/1

== system gm_sampleModel66206_pp_7_1_sub/Subsystem/cfblk136 ==
  emi_42 : Inport  OutDataTypeStr=uint8  PortDimensions=1  SampleTime=1
  Action Port : Inport  Port=2  OutDataTypeStr=boolean  SampleTime=1
  cfblk136 : MinMax
  cfblk136_out1bypassMux : MultiPortSwitch  DataPortOrder=Zero-based contiguous  Inputs=2  zeroidx=on  OutDataTypeStr=uint8  SampleTime=1  SaturateOnIntegerOverflow=off  InputSameDT=off
  emi_43_bypass : UnitDelay  InitialCondition="fi(0,0,8,0,\"hex\",\"00\")"  SampleTime=1
  emi_43 : Outport  SampleTime=1  InitialOutput=0
  wires:
  Action Port/1 -> cfblk136_out1bypassMux/1
  emi_42/1 -> cfblk136/1
  cfblk136/1 -> cfblk136_out1bypassMux/3
  cfblk136_out1bypassMux/1 -> emi_43_bypass/1, emi_43/1
  emi_43_bypass/1 -> cfblk136_out1bypassMux/2

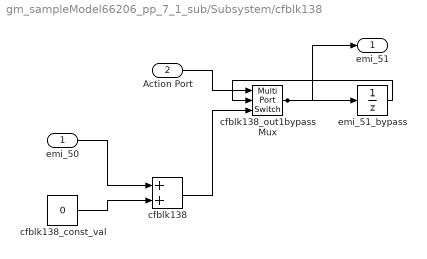
== system gm_sampleModel66206_pp_7_1_sub/Subsystem/cfblk138 ==
  emi_50 : Inport  OutDataTypeStr=uint8  PortDimensions=1  SampleTime=1
  Action Port : Inport  Port=2  OutDataTypeStr=boolean  SampleTime=1
  cfblk138 : Sum  OutDataTypeStr=uint8  AccumDataTypeStr=uint8  RndMeth=Nearest  SampleTime=1
  cfblk138_const_val : Constant  Value=0  VectorParams1D=off  OutDataTypeStr=uint8  SampleTime=1
  cfblk138_out1bypassMux : MultiPortSwitch  DataPortOrder=Zero-based contiguous  Inputs=2  zeroidx=on  OutDataTypeStr=uint8  SampleTime=1  SaturateOnIntegerOverflow=off  InputSameDT=off
  emi_51_bypass : UnitDelay  InitialCondition="fi(0,0,8,0,\"hex\",\"00\")"  SampleTime=1
  emi_51 : Outport  SampleTime=1  InitialOutput=0
  wires:
  Action Port/1 -> cfblk138_out1bypassMux/1
  emi_50/1 -> cfblk138/1
  cfblk138/1 -> cfblk138_out1bypassMux/3
  cfblk138_out1bypassMux/1 -> emi_51_bypass/1, emi_51/1
  emi_51_bypass/1 -> cfblk138_out1bypassMux/2
  cfblk138_const_val/1 -> cfblk138/2

== system gm_sampleModel66206_pp_7_1_sub/Subsystem/cfblk14 ==
  emi_58 : Inport  OutDataTypeStr=uint8  PortDimensions=1  SampleTime=1
  Action Port : Inport  Port=2  OutDataTypeStr=boolean  SampleTime=1
  cfblk14 : simulink/Logic and Bit Operations/Bitwise Operator  logicop=AND  UseBitMask=on  BitMask="fi(0,0,8,0,\"hex\",\"d9\")"  BitMaskRealWorld=Real World Value
  cfblk14_out1bypassMux : MultiPortSwitch  DataPortOrder=Zero-based contiguous  Inputs=2  zeroidx=on  OutDataTypeStr=uint8  SampleTime=1  SaturateOnIntegerOverflow=off  InputSameDT=off
  emi_59_bypass : UnitDelay  InitialCondition="fi(0,0,8,0,\"hex\",\"00\")"  SampleTime=1
  emi_59 : Outport  SampleTime=1  InitialOutput=0
  wires:
  Action Port/1 -> cfblk14_out1bypassMux/1
  emi_58/1 -> cfblk14/1
  cfblk14/1 -> cfblk14_out1bypassMux/3
  cfblk14_out1bypassMux/1 -> emi_59_bypass/1, emi_59/1
  emi_59_bypass/1 -> cfblk14_out1bypassMux/2

== system gm_sampleModel66206_pp_7_1_sub/Subsystem/cfblk146 ==
  In1 : Inport  OutDataTypeStr=uint8  PortDimensions=1  SampleTime=1
  Out1 : Outport  SampleTime=1  InitialOutput=[0]
  wires:
  In1/1 -> Out1/1

== system gm_sampleModel66206_pp_7_1_sub/Subsystem/cfblk147 ==
  In1 : Inport  OutDataTypeStr=uint8  PortDimensions=1  SampleTime=1
  Out1 : Outport  SampleTime=1  InitialOutput=[0]
  wires:
  In1/1 -> Out1/1

== system gm_sampleModel66206_pp_7_1_sub/Subsystem/cfblk148 ==
  In1 : Inport  OutDataTypeStr=uint8  PortDimensions=1  SampleTime=1
  Out1 : Outport  SampleTime=1  InitialOutput=[0]
  wires:
  In1/1 -> Out1/1

== system gm_sampleModel66206_pp_7_1_sub/Subsystem/cfblk149 ==
  In1 : Inport  OutDataTypeStr=uint8  PortDimensions=1  SampleTime=1
  Out1 : Outport  SampleTime=1  InitialOutput=[0]
  wires:
  In1/1 -> Out1/1

== system gm_sampleModel66206_pp_7_1_sub/Subsystem/cfblk150 ==
  In1 : Inport  OutDataTypeStr=uint8  PortDimensions=1  SampleTime=1
  Out1 : Outport  SampleTime=1  InitialOutput=[0]
  wires:
  In1/1 -> Out1/1

== system gm_sampleModel66206_pp_7_1_sub/Subsystem/cfblk151 ==
  In1 : Inport  OutDataTypeStr=uint8  PortDimensions=1  SampleTime=1
  Out1 : Outport  SampleTime=1  InitialOutput=[0]
  wires:
  In1/1 -> Out1/1

== system gm_sampleModel66206_pp_7_1_sub/Subsystem/cfblk168 ==
  emi_90 : Inport  OutDataTypeStr=uint8  PortDimensions=1  SampleTime=1
  Action Port : Inport  Port=2  OutDataTypeStr=boolean  SampleTime=1
  cfblk168 : Subsystem
      settings: MinAlgLoopOccurrences=on
  emi_91 : Outport  SampleTime=1  InitialOutput=0
  wires:
  Action Port/1 -> cfblk168/Enable
  emi_90/1 -> cfblk168/1(in0)
  cfblk168/1(out0) -> emi_91/1

== system gm_sampleModel66206_pp_7_1_sub/Subsystem/cfblk180 ==
  emi_74 : Inport  OutDataTypeStr=uint8  PortDimensions=1  SampleTime=1
  Action Port : Inport  Port=2  OutDataTypeStr=boolean  SampleTime=1
  cfblk180 : DataTypeConversion  OutDataTypeStr=fixdt(0,8,0)
  cfblk180_out1bypassMux : MultiPortSwitch  DataPortOrder=Zero-based contiguous  Inputs=2  zeroidx=on  OutDataTypeStr=uint8  SampleTime=1  SaturateOnIntegerOverflow=off  InputSameDT=off
  emi_75_bypass : UnitDelay  InitialCondition="fi(0,0,8,0,\"hex\",\"00\")"  SampleTime=1
  emi_75 : Outport  SampleTime=1  InitialOutput=0
  wires:
  Action Port/1 -> cfblk180_out1bypassMux/1
  emi_74/1 -> cfblk180/1
  cfblk180/1 -> cfblk180_out1bypassMux/3
  cfblk180_out1bypassMux/1 -> emi_75_bypass/1, emi_75/1
  emi_75_bypass/1 -> cfblk180_out1bypassMux/2

== system gm_sampleModel66206_pp_7_1_sub/Subsystem/cfblk181 ==
  emi_268 : Inport  OutDataTypeStr=uint8  PortDimensions=1  SampleTime=1
  Action Port : Inport  Port=2  OutDataTypeStr=boolean  SampleTime=1
  cfblk181 : DataTypeConversion  OutDataTypeStr=fixdt(0,8,0)
  cfblk181_out1bypassMux : MultiPortSwitch  DataPortOrder=Zero-based contiguous  Inputs=2  zeroidx=on  OutDataTypeStr=uint8  SampleTime=1  SaturateOnIntegerOverflow=off  InputSameDT=off
  emi_269_bypass : UnitDelay  InitialCondition="fi(0,0,8,0,\"hex\",\"00\")"  SampleTime=1
  emi_269 : Outport  SampleTime=1  InitialOutput=0
  wires:
  Action Port/1 -> cfblk181_out1bypassMux/1
  emi_268/1 -> cfblk181/1
  cfblk181/1 -> cfblk181_out1bypassMux/3
  cfblk181_out1bypassMux/1 -> emi_269_bypass/1, emi_269/1
  emi_269_bypass/1 -> cfblk181_out1bypassMux/2

== system gm_sampleModel66206_pp_7_1_sub/Subsystem/cfblk19 ==
  u : Inport  OutDataTypeStr=uint8  SampleTime=1
  FixPt Constant : Constant  DisableCoverage=on  OutDataTypeStr=Inherit: Inherit via back propagation  SampleTime=-1
  FixPt Data Type Duplicate : DataTypeDuplicate  DisableCoverage=on  NumInputPorts=3
  FixPt Sum1 : Sum  OutDataTypeStr=Inherit: Inherit via back propagation  InputSameDT=on  LockScale=on
  y : Outport  SampleTime=1
  wires:
  u/1 -> FixPt Sum1/1, FixPt Data Type Duplicate/2
  FixPt Constant/1 -> FixPt Sum1/2, FixPt Data Type Duplicate/3
  FixPt Sum1/1 -> FixPt Data Type Duplicate/1, y/1

== system gm_sampleModel66206_pp_7_1_sub/Subsystem/cfblk190 ==
  emi_98 : Inport  OutDataTypeStr=uint8  PortDimensions=1  SampleTime=1
  Action Port : Inport  Port=2  OutDataTypeStr=boolean  SampleTime=1
  cfblk190 : DataTypeConversion  OutDataTypeStr=fixdt(0,8,0)
  cfblk190_out1bypassMux : MultiPortSwitch  DataPortOrder=Zero-based contiguous  Inputs=2  zeroidx=on  OutDataTypeStr=uint8  SampleTime=1  SaturateOnIntegerOverflow=off  InputSameDT=off
  emi_99_bypass : UnitDelay  InitialCondition="fi(0,0,8,0,\"hex\",\"00\")"  SampleTime=1
  emi_99 : Outport  SampleTime=1  InitialOutput=0
  wires:
  Action Port/1 -> cfblk190_out1bypassMux/1
  emi_98/1 -> cfblk190/1
  cfblk190/1 -> cfblk190_out1bypassMux/3
  cfblk190_out1bypassMux/1 -> emi_99_bypass/1, emi_99/1
  emi_99_bypass/1 -> cfblk190_out1bypassMux/2

== system gm_sampleModel66206_pp_7_1_sub/Subsystem/cfblk192 ==
  emi_106 : Inport  OutDataTypeStr=uint8  PortDimensions=1  SampleTime=1
  Action Port : Inport  Port=2  OutDataTypeStr=boolean  SampleTime=1
  cfblk192 : DataTypeConversion  OutDataTypeStr=fixdt(0,8,0)
  cfblk192_out1bypassMux : MultiPortSwitch  DataPortOrder=Zero-based contiguous  Inputs=2  zeroidx=on  OutDataTypeStr=uint8  SampleTime=1  SaturateOnIntegerOverflow=off  InputSameDT=off
  emi_107_bypass : UnitDelay  InitialCondition="fi(0,0,8,0,\"hex\",\"00\")"  SampleTime=1
  emi_107 : Outport  SampleTime=1  InitialOutput=0
  wires:
  Action Port/1 -> cfblk192_out1bypassMux/1
  emi_106/1 -> cfblk192/1
  cfblk192/1 -> cfblk192_out1bypassMux/3
  cfblk192_out1bypassMux/1 -> emi_107_bypass/1, emi_107/1
  emi_107_bypass/1 -> cfblk192_out1bypassMux/2

== system gm_sampleModel66206_pp_7_1_sub/Subsystem/cfblk193 ==
  emi_114 : Inport  OutDataTypeStr=uint8  PortDimensions=1  SampleTime=1
  Action Port : Inport  Port=2  OutDataTypeStr=boolean  SampleTime=1
  cfblk193 : DataTypeConversion  OutDataTypeStr=fixdt(0,8,0)
  cfblk193_out1bypassMux : MultiPortSwitch  DataPortOrder=Zero-based contiguous  Inputs=2  zeroidx=on  OutDataTypeStr=uint8  SampleTime=1  SaturateOnIntegerOverflow=off  InputSameDT=off
  emi_115_bypass : UnitDelay  InitialCondition="fi(0,0,8,0,\"hex\",\"00\")"  SampleTime=1
  emi_115 : Outport  SampleTime=1  InitialOutput=0
  wires:
  Action Port/1 -> cfblk193_out1bypassMux/1
  emi_114/1 -> cfblk193/1
  cfblk193/1 -> cfblk193_out1bypassMux/3
  cfblk193_out1bypassMux/1 -> emi_115_bypass/1, emi_115/1
  emi_115_bypass/1 -> cfblk193_out1bypassMux/2

== system gm_sampleModel66206_pp_7_1_sub/Subsystem/cfblk2 ==
  emi_194 : Inport  OutDataTypeStr=uint8  PortDimensions=1  SampleTime=1
  Action Port : Inport  Port=2  OutDataTypeStr=boolean  SampleTime=1
  cfblk2 : Subsystem  mask(Detect Increase){vinit=double(0), InputProcessing=Elements as channels (sample based), OutDataTypeStr=uint8}
      mask prompts: vinit "Simulink:masks:InitialCondition_MP"; InputProcessing "Simulink:masks:InputProcessing_MP"; OutDataTypeStr "Simulink:masks:OutputDataType_MP"
      mask help: Simulink:masks:DetectIncrease_MD
      mask TypeOptions InputProcessing: Simulink:masks:ColumnsAsChannelsFrameBased | Simulink:masks:ElementsAsChannelsSampleBased
      mask TypeOptions OutDataTypeStr: Simulink:masks:uint8 | Simulink:masks:boolean
      mask Display: fprintf('U > U/z')
  cfblk2_out1bypassMux : MultiPortSwitch  DataPortOrder=Zero-based contiguous  Inputs=2  zeroidx=on  OutDataTypeStr=uint8  SampleTime=1  SaturateOnIntegerOverflow=off  InputSameDT=off
  emi_195_bypass : UnitDelay  InitialCondition="fi(0,0,8,0,\"hex\",\"00\")"  SampleTime=1
  emi_195 : Outport  SampleTime=1  InitialOutput=0
  wires:
  Action Port/1 -> cfblk2_out1bypassMux/1, cfblk2/2(Action Port_out2)
  emi_194/1 -> cfblk2/1(U)
  cfblk2/1(Y) -> cfblk2_out1bypassMux/3
  cfblk2_out1bypassMux/1 -> emi_195_bypass/1, emi_195/1
  emi_195_bypass/1 -> cfblk2_out1bypassMux/2

== system gm_sampleModel66206_pp_7_1_sub/Subsystem/cfblk20_inst ==
  in1 : Inport  OutDataTypeStr=uint8  SampleTime=1
  in2 : Inport  Port=2  OutDataTypeStr=uint8  SampleTime=1
  mul_cfblk20_dotp_mulcomp : Product  Inputs=**  OutDataTypeStr=uint8  SampleTime=1
  out1 : Outport  OutDataTypeStr=uint8  SampleTime=1
  wires:
  in1/1 -> mul_cfblk20_dotp_mulcomp/1
  in2/1 -> mul_cfblk20_dotp_mulcomp/2
  mul_cfblk20_dotp_mulcomp/1 -> out1/1

== system gm_sampleModel66206_pp_7_1_sub/Subsystem/cfblk21 ==
  emi_122 : Inport  OutDataTypeStr=uint8  PortDimensions=1  SampleTime=1
  Action Port : Inport  Port=2  OutDataTypeStr=boolean  SampleTime=1
  cfblk21 : Subsystem  mask(Real World Value Increment){}
      mask help: Simulink:masks:RealWorldValueIncrement_MD
      mask Display: disp('V++')
  cfblk21_out1bypassMux : MultiPortSwitch  DataPortOrder=Zero-based contiguous  Inputs=2  zeroidx=on  OutDataTypeStr=uint8  SampleTime=1  SaturateOnIntegerOverflow=off  InputSameDT=off
  emi_123_bypass : UnitDelay  InitialCondition="fi(0,0,8,0,\"hex\",\"00\")"  SampleTime=1
  emi_123 : Outport  SampleTime=1  InitialOutput=0
  wires:
  Action Port/1 -> cfblk21_out1bypassMux/1
  emi_122/1 -> cfblk21/1(u)
  cfblk21/1(y) -> cfblk21_out1bypassMux/3
  cfblk21_out1bypassMux/1 -> emi_123_bypass/1, emi_123/1
  emi_123_bypass/1 -> cfblk21_out1bypassMux/2

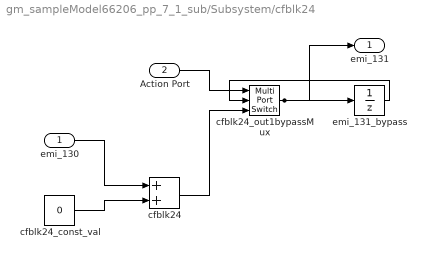
== system gm_sampleModel66206_pp_7_1_sub/Subsystem/cfblk24 ==
  emi_130 : Inport  OutDataTypeStr=uint8  PortDimensions=1  SampleTime=1
  Action Port : Inport  Port=2  OutDataTypeStr=boolean  SampleTime=1
  cfblk24 : Sum  OutDataTypeStr=uint8  AccumDataTypeStr=uint8  RndMeth=Nearest  SampleTime=1
  cfblk24_const_val : Constant  Value=0  VectorParams1D=off  OutDataTypeStr=uint8  SampleTime=1
  cfblk24_out1bypassMux : MultiPortSwitch  DataPortOrder=Zero-based contiguous  Inputs=2  zeroidx=on  OutDataTypeStr=uint8  SampleTime=1  SaturateOnIntegerOverflow=off  InputSameDT=off
  emi_131_bypass : UnitDelay  InitialCondition="fi(0,0,8,0,\"hex\",\"00\")"  SampleTime=1
  emi_131 : Outport  SampleTime=1  InitialOutput=0
  wires:
  Action Port/1 -> cfblk24_out1bypassMux/1
  emi_130/1 -> cfblk24/1
  cfblk24/1 -> cfblk24_out1bypassMux/3
  cfblk24_out1bypassMux/1 -> emi_131_bypass/1, emi_131/1
  emi_131_bypass/1 -> cfblk24_out1bypassMux/2
  cfblk24_const_val/1 -> cfblk24/2

== system gm_sampleModel66206_pp_7_1_sub/Subsystem/cfblk26 ==
  emi_138 : Inport  OutDataTypeStr=uint8  PortDimensions=1  SampleTime=1
  Action Port : Inport  Port=2  OutDataTypeStr=boolean  SampleTime=1
  cfblk26 : Gain  Gain="fi(0,0,8,7,\"hex\",\"80\")"  ParamDataTypeStr=fixdt(0, 8, 7)  OutDataTypeStr=fixdt(0, 16, 7)  SampleTime=1
  cfblk26_out1bypassMux : MultiPortSwitch  DataPortOrder=Zero-based contiguous  Inputs=2  zeroidx=on  OutDataTypeStr=fixdt(0, 16, 7)  SampleTime=1  SaturateOnIntegerOverflow=off  InputSameDT=off
  emi_139_bypass : UnitDelay  InitialCondition="fi(0,0,16,7,\"hex\",\"0000\")"  SampleTime=1
  emi_139 : Outport  SampleTime=1  InitialOutput=0
  wires:
  Action Port/1 -> cfblk26_out1bypassMux/1
  emi_138/1 -> cfblk26/1
  cfblk26/1 -> cfblk26_out1bypassMux/3
  cfblk26_out1bypassMux/1 -> emi_139_bypass/1, emi_139/1
  emi_139_bypass/1 -> cfblk26_out1bypassMux/2

== system gm_sampleModel66206_pp_7_1_sub/Subsystem/cfblk27 ==
  emi_146 : Inport  OutDataTypeStr=uint8  PortDimensions=1  SampleTime=1
  Action Port : Inport  Port=2  OutDataTypeStr=boolean  SampleTime=1
  cfblk27 : Sum  Inputs=+
  cfblk27_out1bypassMux : MultiPortSwitch  DataPortOrder=Zero-based contiguous  Inputs=2  zeroidx=on  OutDataTypeStr=uint8  SampleTime=1  SaturateOnIntegerOverflow=off  InputSameDT=off
  emi_147_bypass : UnitDelay  InitialCondition="fi(0,0,8,0,\"hex\",\"00\")"  SampleTime=1
  emi_147 : Outport  SampleTime=1  InitialOutput=0
  wires:
  Action Port/1 -> cfblk27_out1bypassMux/1
  emi_146/1 -> cfblk27/1
  cfblk27/1 -> cfblk27_out1bypassMux/3
  cfblk27_out1bypassMux/1 -> emi_147_bypass/1, emi_147/1
  emi_147_bypass/1 -> cfblk27_out1bypassMux/2

== system gm_sampleModel66206_pp_7_1_sub/Subsystem/cfblk28 ==
  emi_154 : Inport  OutDataTypeStr=uint8  PortDimensions=1  SampleTime=1
  Action Port : Inport  Port=2  OutDataTypeStr=boolean  SampleTime=1
  cfblk28 : Subsystem  mask(Real World Value Increment){}
      mask help: Simulink:masks:RealWorldValueIncrement_MD
      mask Display: disp('V++')
  cfblk28_out1bypassMux : MultiPortSwitch  DataPortOrder=Zero-based contiguous  Inputs=2  zeroidx=on  OutDataTypeStr=uint8  SampleTime=1  SaturateOnIntegerOverflow=off  InputSameDT=off
  emi_155_bypass : UnitDelay  InitialCondition="fi(0,0,8,0,\"hex\",\"00\")"  SampleTime=1
  emi_155 : Outport  SampleTime=1  InitialOutput=0
  wires:
  Action Port/1 -> cfblk28_out1bypassMux/1
  emi_154/1 -> cfblk28/1(u)
  cfblk28/1(y) -> cfblk28_out1bypassMux/3
  cfblk28_out1bypassMux/1 -> emi_155_bypass/1, emi_155/1
  emi_155_bypass/1 -> cfblk28_out1bypassMux/2

== system gm_sampleModel66206_pp_7_1_sub/Subsystem/cfblk30_inst ==
  in1 : Inport  OutDataTypeStr=uint8  SampleTime=1
  in2 : Inport  Port=2  OutDataTypeStr=uint8  SampleTime=1
  mul_cfblk30_dotp_mulcomp : Product  Inputs=**  OutDataTypeStr=uint8  SampleTime=1
  out1 : Outport  OutDataTypeStr=uint8  SampleTime=1
  wires:
  in1/1 -> mul_cfblk30_dotp_mulcomp/1
  in2/1 -> mul_cfblk30_dotp_mulcomp/2
  mul_cfblk30_dotp_mulcomp/1 -> out1/1

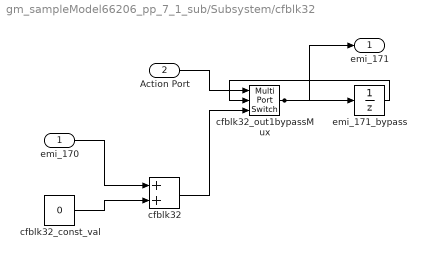
== system gm_sampleModel66206_pp_7_1_sub/Subsystem/cfblk32 ==
  emi_170 : Inport  OutDataTypeStr=uint8  PortDimensions=1  SampleTime=1
  Action Port : Inport  Port=2  OutDataTypeStr=boolean  SampleTime=1
  cfblk32 : Sum  OutDataTypeStr=uint8  AccumDataTypeStr=uint8  RndMeth=Nearest  SampleTime=1
  cfblk32_const_val : Constant  Value=0  VectorParams1D=off  OutDataTypeStr=uint8  SampleTime=1
  cfblk32_out1bypassMux : MultiPortSwitch  DataPortOrder=Zero-based contiguous  Inputs=2  zeroidx=on  OutDataTypeStr=uint8  SampleTime=1  SaturateOnIntegerOverflow=off  InputSameDT=off
  emi_171_bypass : UnitDelay  InitialCondition="fi(0,0,8,0,\"hex\",\"00\")"  SampleTime=1
  emi_171 : Outport  SampleTime=1  InitialOutput=0
  wires:
  Action Port/1 -> cfblk32_out1bypassMux/1
  emi_170/1 -> cfblk32/1
  cfblk32/1 -> cfblk32_out1bypassMux/3
  cfblk32_out1bypassMux/1 -> emi_171_bypass/1, emi_171/1
  emi_171_bypass/1 -> cfblk32_out1bypassMux/2
  cfblk32_const_val/1 -> cfblk32/2
